simulink model "vertical_smm_with_lqr_2d"  (R2015a)
settings: Solver=FixedStepDiscrete  StartTime=0.0  StopTime=inf  FixedStep=sample_time  RelTol=1e-3
undefined symbols (not defined in the file or in its folder): A_kalman_fourbar_gear, A_kalman_transverse, A_kalman_vertical, A_lpf_dtau, A_lpf_leg_spring, B1_lpf_dtau, B1_lpf_leg_spring, B2_lpf_dtau, B2_lpf_leg_spring, B_dx_versus_x0, B_kalman_fourbar_gear, B_kalman_transverse, B_kalman_vertical, backwards_K_sag_of_t, boom_mount_angle, C_kalman_fourbar_gear, C_kalman_transverse, C_kalman_vertical, com_leg_motor, com_torso, contact_threshold, control_start_time, d_vertical_boom_com_offset, d_vertical_com, desired_com_forward_velocity, desired_torso_angle, Discrete, fcut_contact, forward_dx, forward_dx_of_dxstar, forward_velocity_target_step, forward_x, forward_x_of_dxstar, g, h_boom, HIP_MTR_MAX_CONT_TORQUE, i_robot, initial_dx_estimate, initial_dy_estimate, initial_dz_estimate, initial_z_estimate, j_leg, j_motor, j_segments, k_LQR_vertical, k_sea, k_vertical_winch, kalman_load_to_deflect_transmission, kalman_stance_slip_threshold, kd_lateral, kd_motor, kp_lateral, kp_motor, l_boom_projected, l_retract_delta, l_retract_swing_max, l_retract_swing_min, l_seg, lambda1, lambda2 ... (+60)
libraries: simulink x9, ctrlSharedLib x7
(part 2 of 4)

== system vertical_smm_with_lqr_2d/Control/Behavior Control/R Leg Calculator ==
  Front [rad rad/s] : Inport
  Back [rad rad/s] : Inport  Port=2
  Demux1 : Demux  Outputs=2
  Gain1 : Gain  Gain=2*l_seg
  Gain2 : Gain  Gain=l_seg
  Gain3 : Gain  Gain=-1
  Gain4 : Gain  Gain=0.5
  Gain5 : Gain  Gain=0.5
  Gain6 : Gain  Gain=2
  Mux1 : Mux  Inputs=2
  Product : Product  RndMeth=Zero
  Sum4 : Sum  Inputs=+|+
  Sum5 : Sum  Inputs=+|-
  Trigonometric Function : Trigonometry  Operator=cos
  Trigonometric Function1 : Trigonometry
  "Leg Length [m m/s] " : Outport
  Leg Angle [rad rad/s] : Outport  Port=2
  Leg Splay [rad rad/s] : Outport  Port=3
  w [m] : Outport  Port=4
  wires:
  Gain5/1 -> Leg Angle [rad rad/s]/1
  Sum4/1 -> Gain5/1
  Mux1/1 -> "Leg Length [m m/s] "/1
  Sum5/1 -> Demux1/1, Leg Splay [rad rad/s]/1
  Gain2/1 -> Gain6/1, Product/1
  Demux1/1 -> Gain4/1
  Gain3/1 -> Product/2
  Demux1/2 -> Gain3/1
  Back [rad rad/s]/1 -> Sum5/1, Sum4/1
  Front [rad rad/s]/1 -> Sum4/2, Sum5/2
  Product/1 -> Mux1/2
  Trigonometric Function1/1 -> Gain2/1
  Gain1/1 -> Mux1/1
  Trigonometric Function/1 -> Gain1/1
  Gain4/1 -> Trigonometric Function/1, Trigonometric Function1/1
  Gain6/1 -> w [m]/1

== system vertical_smm_with_lqr_2d/Control/Behavior Control/Secondary Leg Behavior ==
  note: Mirror the primary
      | leg motion
  note: Position control the
      | individual four bar segments
  note: Convert to
      | four-bar angles
  Secondary Back Gear [rad rad/s] : Inport
  Secondary Front Gear [rad rad/s] : Inport  Port=2
  Torso Pitch [rad rad/s] : Inport  Port=3
  Right/Left Secondary [1/0] : Inport  Port=4
  Primary Leg Angle [rad rad/s] : Inport  Port=5
  Primary Leg Length [m m/s] : Inport  Port=6
  Avoid Hitting Mechanical Limits : MATLAB Function  TreatAsAtomicUnit=on
  Back/Front Motor PD : Subsystem
  Constant4 : Constant  Value=0
  Constant5 : Constant  Value=0  OutDataTypeStr=boolean
  Demux{1..3,5} (4 alike) : Demux  Outputs=2
  Demux6 : Demux  Outputs=6
  Fcn2 : Fcn  Expr=2*pi-u(1)
  Mirrored Leg Length Target : MATLAB Function  TreatAsAtomicUnit=on
  Mux{1..4,7,11} (6 alike) : Mux  Inputs=2
  Mux5 : Mux  Inputs=3
  Mux6 : Mux  Inputs=3
  Sum1 : Sum  Inputs=++|
  Virtual Leg to Four Bar : MATLAB Function  TreatAsAtomicUnit=on
  k_virtual6 : Gain  Gain=-1
  two_pole_filter : DiscreteTransferFcn  Numerator=[A_lpf_leg_spring 0 0]  Denominator=[1 B1_lpf_leg_spring B2_lpf_leg_spring]  SampleTime=sample_time
  Secondary Back/Front Motor Torque [Nm Nm] : Outport
  Secondary Force or Position Control [1/0] : Outport  Port=2
  wires:
  Constant5/1 -> Secondary Force or Position Control [1/0]/1
  Back/Front Motor PD/1(Commanded Torque [Nm] [back front]) -> Secondary Back/Front Motor Torque [Nm Nm]/1
  Demux5/2 -> k_virtual6/1
  Demux5/1 -> Fcn2/1
  Primary Leg Angle [rad rad/s]/1 -> two_pole_filter/1
  Mirrored Leg Length Target/2(dl_leg) -> Mux5/2
  Mirrored Leg Length Target/3(ddl_leg) -> Mux5/3
  Mirrored Leg Length Target/1(l_leg) -> Mux5/1
  Constant4/1 -> Mux6/3
  k_virtual6/1 -> Mux6/2
  Fcn2/1 -> Mux6/1
  Mux7/1 -> Demux6/1
  Torso Pitch [rad rad/s]/1 -> Sum1/1
  Mux5/1 -> Mux7/1
  Mux6/1 -> Mux7/2
  Virtual Leg to Four Bar/1(back) -> Avoid Hitting Mechanical Limits/1(back_desired)
  Virtual Leg to Four Bar/2(dback) -> Avoid Hitting Mechanical Limits/2(dback_desired)
  Virtual Leg to Four Bar/3(ddback) -> Avoid Hitting Mechanical Limits/3(ddback_desired)
  Virtual Leg to Four Bar/4(front) -> Avoid Hitting Mechanical Limits/4(front_desired)
  Virtual Leg to Four Bar/5(dfront) -> Avoid Hitting Mechanical Limits/5(dfront_desired)
  Virtual Leg to Four Bar/6(ddfront) -> Avoid Hitting Mechanical Limits/6(ddfront_desired)
  Demux6/1 -> Virtual Leg to Four Bar/1(l_leg)
  Demux6/2 -> Virtual Leg to Four Bar/2(dl_leg)
  Demux6/3 -> Virtual Leg to Four Bar/3(ddl_leg)
  Demux6/4 -> Virtual Leg to Four Bar/4(phi)
  Demux6/5 -> Virtual Leg to Four Bar/5(dphi)
  Demux6/6 -> Virtual Leg to Four Bar/6(ddphi)
  Mux11/1 -> Back/Front Motor PD/5(Measured Velocity [rad/s] [back front])
  Demux2/2 -> Mux11/2
  Mux4/1 -> Back/Front Motor PD/4(Measured Position [rad] [back front])
  Mux1/1 -> Back/Front Motor PD/1(Desired Position [rad] [back front])
  Right/Left Secondary [1/0]/1 -> Back/Front Motor PD/6(Right/Left Leg [1/0])
  Demux3/2 -> Mux11/1
  Demux3/1 -> Mux4/1
  Avoid Hitting Mechanical Limits/2(front_cmd) -> Mux1/2
  Avoid Hitting Mechanical Limits/1(back_cmd) -> Mux1/1
  Demux2/1 -> Mux4/2
  Secondary Front Gear [rad rad/s]/1 -> Demux2/1
  Secondary Back Gear [rad rad/s]/1 -> Demux3/1
  Avoid Hitting Mechanical Limits/3(dback_cmd) -> Mux2/1
  Avoid Hitting Mechanical Limits/4(dfront_cmd) -> Mux2/2
  Avoid Hitting Mechanical Limits/5(ddback_cmd) -> Mux3/1
  Avoid Hitting Mechanical Limits/6(ddfront_cmd) -> Mux3/2
  Mux2/1 -> Back/Front Motor PD/2(Desired Velocity [rad/s] [back front])
  Mux3/1 -> Back/Front Motor PD/3(Desired Acceleration [rad/s^2] [back front])
  two_pole_filter/1 -> Sum1/2
  Sum1/1 -> Demux5/1
  Demux1/1 -> Mirrored Leg Length Target/1(primary_l_leg)
  Demux1/2 -> Mirrored Leg Length Target/2(primary_dl_leg)
  Primary Leg Length [m m/s]/1 -> Demux1/1

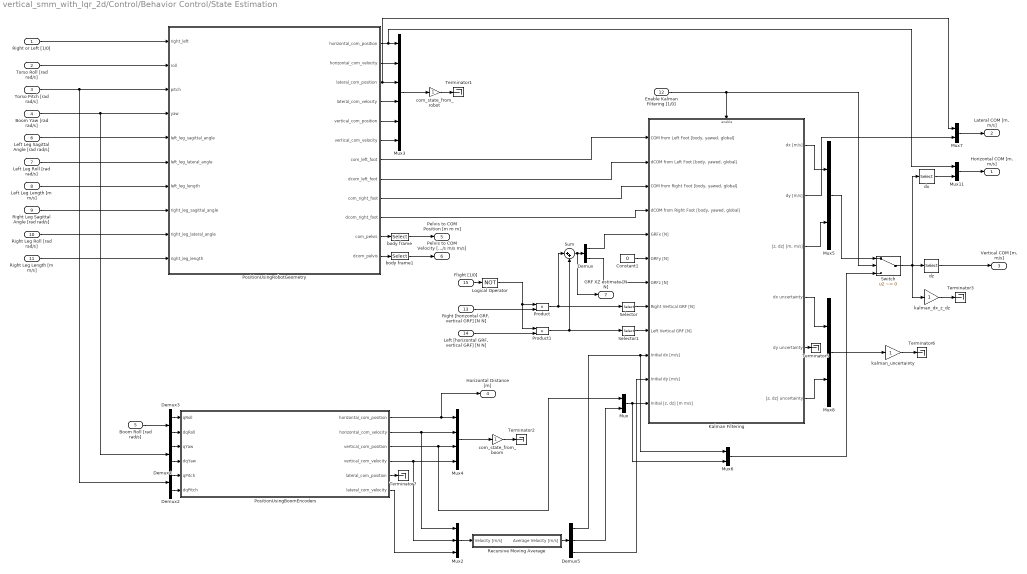
== system vertical_smm_with_lqr_2d/Control/Behavior Control/State Estimation ==
  Right or Left [1/0] : Inport
  Torso Roll [rad rad/s] : Inport  Port=2
  Torso Pitch [rad rad/s] : Inport  Port=3
  Boom Yaw [rad rad/s] : Inport  Port=4
  Boom Roll [rad rad/s] : Inport  Port=5
  Left Leg Sagittal Angle [rad rad/s] : Inport  Port=6
  Left Leg Roll [rad rad/s] : Inport  Port=7
  Left Leg Length [m m/s] : Inport  Port=8
  Right Leg Sagittal Angle [rad rad/s] : Inport  Port=9
  Right Leg Roll [rad rad/s] : Inport  Port=10
  Right Leg Length [m m/s] : Inport  Port=11
  Enable Kalman Filtering [1/0] : Inport  Port=12
  "Right [horizontal GRF, vertical GRF] [N N]" : Inport  Port=13
  "Left [horizontal GRF, vertical GRF] [N N]" : Inport  Port=14
  Flight [1/0] : Inport  Port=15
  Constant1 : Constant  Value=0
  Demux{,2..4} (4 alike) : Demux  Outputs=2
  Demux5 : Demux  Outputs=3
  Kalman Filtering : Subsystem
  Logical Operator : Logic  Operator=NOT  AllPortsSameDT=off  OutDataTypeStr=boolean
  Mux{,5..8,11} (6 alike) : Mux  Inputs=2
  Mux2 : Mux  Inputs=3
  Mux3 : Mux  Inputs=6
  Mux4 : Mux
  PositionUsingBoomEncoders : MATLAB Function  TreatAsAtomicUnit=on
  PositionUsingRobotGeometry : MATLAB Function  TreatAsAtomicUnit=on
  Product : Product
  Product1 : Product
  Recursive Moving Average : Subsystem
  Selector : Selector  InputPortWidth=2  Indices=[2]
  Selector1 : Selector  InputPortWidth=2  Indices=[2]
  Sum : Sum  Inputs=|++
  Switch : Switch  Criteria=u2 ~= 0
  Terminator{1..3,5..7} (6 alike) : Terminator
  body frame : Selector  InputPortWidth=9  Indices=[1 2 3]
  body frame1 : Selector  InputPortWidth=9  Indices=[1 2 3]
  com_state_from_boom : Gain
  com_state_from_robot : Gain
  dx : Selector  InputPortWidth=3  Indices=[1]
  dz : Selector  InputPortWidth=3  Indices=[2 3]
  kalman_dx_z_dz : Gain
  kalman_uncertainty : Gain
  "Horizontal COM [m, m/s]" : Outport
  "Lateral COM [m, m/s]" : Outport  Port=2
  "Vertical COM [m, m/s]" : Outport  Port=3
  Horizontal Distance [m] : Outport  Port=4
  Pelvis to COM Position [m m m] : Outport  Port=5
  Pelvis to COM Velocity [m/s m/s m/s] : Outport  Port=6
  GRF XZ estimate [N N] : Outport  Port=7
  wires:
  com_state_from_boom/1 -> Terminator2/1
  Kalman Filtering/1(dx [m/s]) -> Mux5/1
  Demux2/1 -> PositionUsingBoomEncoders/5(qPitch)
  Demux2/2 -> PositionUsingBoomEncoders/6(dqPitch)
  Mux3/1 -> com_state_from_robot/1
  com_state_from_robot/1 -> Terminator1/1
  PositionUsingRobotGeometry/1(horizontal_com_position) -> Mux3/1, Mux11/1
  PositionUsingBoomEncoders/1(horizontal_com_position) -> Horizontal Distance [m]/1, Mux4/1
  PositionUsingBoomEncoders/3(vertical_com_position) -> Mux/1, Mux4/3
  PositionUsingBoomEncoders/4(vertical_com_velocity) -> Mux2/2, Mux4/4
  Mux4/1 -> com_state_from_boom/1
  Left Leg Sagittal Angle [rad rad/s]/1 -> PositionUsingRobotGeometry/5(left_leg_sagittal_angle)
  Left Leg Roll [rad rad/s]/1 -> PositionUsingRobotGeometry/6(left_leg_lateral_angle)
  Left Leg Length [m m/s]/1 -> PositionUsingRobotGeometry/7(left_leg_length)
  Right Leg Sagittal Angle [rad rad/s]/1 -> PositionUsingRobotGeometry/8(right_leg_sagittal_angle)
  Right Leg Roll [rad rad/s]/1 -> PositionUsingRobotGeometry/9(right_leg_lateral_angle)
  Right Leg Length [m m/s]/1 -> PositionUsingRobotGeometry/10(right_leg_length)
  Right or Left [1/0]/1 -> PositionUsingRobotGeometry/1(right_left)
  Torso Roll [rad rad/s]/1 -> PositionUsingRobotGeometry/2(roll)
  Boom Yaw [rad rad/s]/1 -> Demux4/1, PositionUsingRobotGeometry/4(yaw)
  Torso Pitch [rad rad/s]/1 -> Demux2/1, PositionUsingRobotGeometry/3(pitch)
  Demux3/2 -> PositionUsingBoomEncoders/2(dqRoll)
  Demux3/1 -> PositionUsingBoomEncoders/1(qRoll)
  Boom Roll [rad rad/s]/1 -> Demux3/1
  Demux4/1 -> PositionUsingBoomEncoders/3(qYaw)
  Demux4/2 -> PositionUsingBoomEncoders/4(dqYaw)
  PositionUsingRobotGeometry/7(com_left_foot) -> Kalman Filtering/1("COM from Left Foot [body, yawed, global]")
  PositionUsingRobotGeometry/8(dcom_left_foot) -> Kalman Filtering/2("dCOM from Left Foot [body, yawed, global]")
  PositionUsingRobotGeometry/9(com_right_foot) -> Kalman Filtering/3("COM from Right Foot [body, yawed, global]")
  PositionUsingRobotGeometry/10(dcom_right_foot) -> Kalman Filtering/4("dCOM from Right Foot [body, yawed, global]")
  Kalman Filtering/2(dy [m/s]) -> Mux7/2
  Kalman Filtering/3("[z, dz] [m, m/s]") -> Mux5/2
  Mux2/1 -> Recursive Moving Average/1(Velocity [m/s])
  dx/1 -> Mux11/2
  Mux5/1 -> Switch/1
  Constant1/1 -> Kalman Filtering/6(GRFy [N])
  Recursive Moving Average/1(Average Velocity [m/s]) -> Demux5/1
  Mux/1 -> Mux6/2, Kalman Filtering/12("Initial [z, dz] [m m/s]")
  Demux5/2 -> Mux/2
  PositionUsingBoomEncoders/2(horizontal_com_velocity) -> Mux2/1, Mux4/2
  Selector/1 -> Kalman Filtering/8(Right Vertical GRF [N])
  Selector1/1 -> Kalman Filtering/9(Left Vertical GRF [N])
  Product1/1 -> Sum/2, Selector1/1
  Product/1 -> Sum/1, Selector/1
  Sum/1 -> GRF XZ estimate [N N]/1, Demux/1
  Enable Kalman Filtering [1/0]/1 -> Switch/2, Kalman Filtering/Enable
  kalman_dx_z_dz/1 -> Terminator3/1
  Demux5/1 -> Mux6/1, Kalman Filtering/10(Initial dx [m/s])
  Demux/1 -> Kalman Filtering/5(GRFx [N])
  Demux/2 -> Kalman Filtering/7(GRFz [N])
  Flight [1/0]/1 -> Logical Operator/1
  "Right [horizontal GRF, vertical GRF] [N N]"/1 -> Product/2
  Logical Operator/1 -> Product1/1, Product/1
  "Left [horizontal GRF, vertical GRF] [N N]"/1 -> Product1/2
  Kalman Filtering/4(dx uncertainty) -> Mux8/1
  Kalman Filtering/6("[z, dz] uncertainty") -> Mux8/2
  Kalman Filtering/5(dy uncertainty) -> Terminator5/1
  kalman_uncertainty/1 -> Terminator6/1
  Mux8/1 -> kalman_uncertainty/1
  PositionUsingRobotGeometry/12(dcom_pelvis) -> body frame1/1
  PositionUsingRobotGeometry/11(com_pelvis) -> body frame/1
  Mux11/1 -> "Horizontal COM [m, m/s]"/1
  body frame/1 -> Pelvis to COM Position [m m m]/1
  body frame1/1 -> Pelvis to COM Velocity [m/s m/s m/s]/1
  PositionUsingRobotGeometry/6(vertical_com_velocity) -> Mux3/6
  PositionUsingRobotGeometry/5(vertical_com_position) -> Mux3/5
  PositionUsingRobotGeometry/4(lateral_com_velocity) -> Mux3/4
  PositionUsingRobotGeometry/3(lateral_com_position) -> Mux3/3, Mux7/1
  PositionUsingRobotGeometry/2(horizontal_com_velocity) -> Mux3/2
  Mux6/1 -> Switch/3
  dz/1 -> "Vertical COM [m, m/s]"/1
  Switch/1 -> dx/1, dz/1, kalman_dx_z_dz/1
  Mux7/1 -> "Lateral COM [m, m/s]"/1
  PositionUsingBoomEncoders/5(lateral_com_position) -> Terminator7/1
  PositionUsingBoomEncoders/6(lateral_com_velocity) -> Mux2/3
  Demux5/3 -> Kalman Filtering/11(Initial dy [m/s])

== system vertical_smm_with_lqr_2d/Control/Behavior Control/Torque Distribution Left ==
  Leg Torque [Nm] : Inport
  Leg Force [N] : Inport  Port=2
  w [m] : Inport  Port=3
  Gain : Gain  Gain=0.5
  Gain1 : Gain  Gain=0.5
  Motor Torque Saturation Optimization : MATLAB Function  TreatAsAtomicUnit=on
  Product : Product  RndMeth=Zero
  Sum : Sum  Inputs=|++
  Sum1 : Sum  Inputs=+-|
  Back Torque [Nm] : Outport
  Front Torque [Nm] : Outport  Port=2
  wires:
  Gain/1 -> Motor Torque Saturation Optimization/1(x1s)
  Gain1/1 -> Motor Torque Saturation Optimization/2(x2s)
  Product/1 -> Gain1/1
  Leg Force [N]/1 -> Product/1
  Motor Torque Saturation Optimization/2(t2) -> Sum/2, Sum1/2
  w [m]/1 -> Product/2
  Motor Torque Saturation Optimization/1(t1) -> Sum1/1, Sum/1
  Sum/1 -> Front Torque [Nm]/1
  Leg Torque [Nm]/1 -> Gain/1
  Sum1/1 -> Back Torque [Nm]/1

== system vertical_smm_with_lqr_2d/Control/Behavior Control/Torque Distribution Right ==
  Leg Torque [Nm] : Inport
  Leg Force [N] : Inport  Port=2
  w [m] : Inport  Port=3
  Gain : Gain  Gain=0.5
  Gain1 : Gain  Gain=0.5
  Motor Torque Saturation Optimization : MATLAB Function  TreatAsAtomicUnit=on
  Product : Product  RndMeth=Zero
  Sum : Sum  Inputs=|++
  Sum1 : Sum  Inputs=+-|
  Back Torque [Nm] : Outport
  Front Torque [Nm] : Outport  Port=2
  wires:
  Sum1/1 -> Back Torque [Nm]/1
  Leg Torque [Nm]/1 -> Gain/1
  Sum/1 -> Front Torque [Nm]/1
  Motor Torque Saturation Optimization/1(t1) -> Sum/1, Sum1/1
  w [m]/1 -> Product/2
  Motor Torque Saturation Optimization/2(t2) -> Sum1/2, Sum/2
  Leg Force [N]/1 -> Product/1
  Product/1 -> Gain1/1
  Gain1/1 -> Motor Torque Saturation Optimization/2(x2s)
  Gain/1 -> Motor Torque Saturation Optimization/1(x1s)

== system vertical_smm_with_lqr_2d/Control/Behavior Control/dtau_des ==
  x : Inport
  Gain1 : Gain  Gain=1/sample_time
  difference : simulink/Discrete/Difference  ICPrevInput=0.0  InputProcessing=Inherited  OutMin=[]  OutMax=[]  OutDataType=fixdt(1, 16)  OutScaling=2^-10  DoSatur=off
  two_pole_filter : DiscreteTransferFcn  Numerator=[A_lpf_dtau 0 0]  Denominator=[1 B1_lpf_dtau B2_lpf_dtau]  SampleTime=sample_time
  dx/dt : Outport
  wires:
  two_pole_filter/1 -> dx/dt/1
  x/1 -> Gain1/1
  difference/1 -> two_pole_filter/1
  Gain1/1 -> difference/1

== system vertical_smm_with_lqr_2d/Control/Behavior Control/Force Estimation/Horizontal GRF ==
  Axial Force [N] : Inport
  Orthogonal Force [N] : Inport  Port=2
  Torso Pitch [rad] : Inport  Port=3
  Leg Angle [rad] : Inport  Port=4
  Gain : Gain  Gain=-1
  Gain1 : Gain  Gain=-1
  Product : Product
  Product1 : Product
  Sum : Sum  Inputs=++|
  Sum1 : Sum  Inputs=+|+
  Trigonometric Function : Trigonometry
  Trigonometric Function1 : Trigonometry  Operator=cos
  Horizontal Force [N] : Outport
  wires:
  Product1/1 -> Gain/1
  Sum1/1 -> Horizontal Force [N]/1
  Trigonometric Function1/1 -> Product1/2
  Orthogonal Force [N]/1 -> Product1/1
  Axial Force [N]/1 -> Product/1
  Leg Angle [rad]/1 -> Sum/2
  Torso Pitch [rad]/1 -> Sum/1
  Trigonometric Function/1 -> Product/2
  Sum/1 -> Trigonometric Function/1, Trigonometric Function1/1
  Product/1 -> Gain1/1
  Gain/1 -> Sum1/2
  Gain1/1 -> Sum1/1

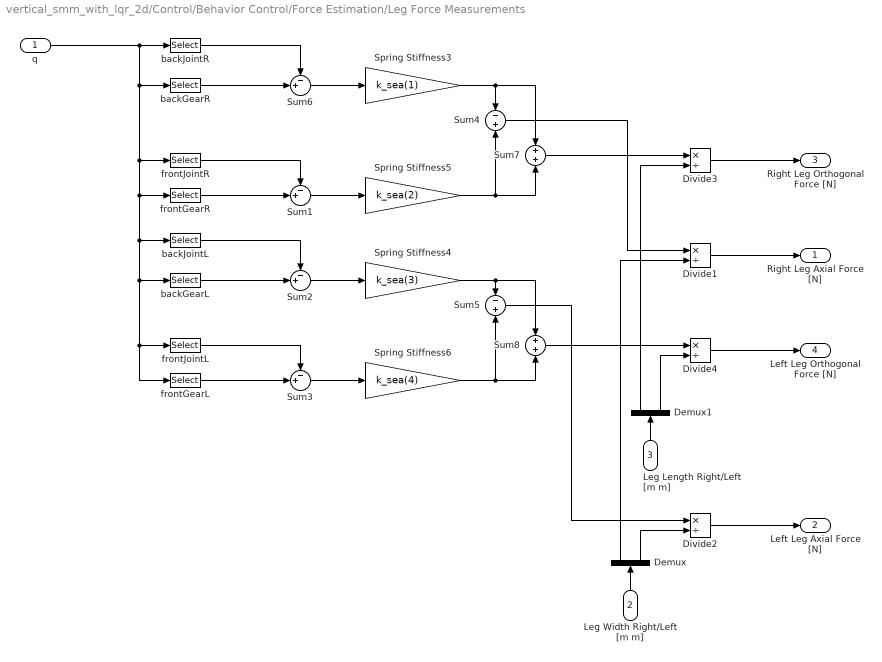
== system vertical_smm_with_lqr_2d/Control/Behavior Control/Force Estimation/Leg Force Measurements ==
  q : Inport
  Leg Width Right/Left [m m] : Inport  Port=2
  Leg Length Right/Left [m m] : Inport  Port=3
  Demux : Demux  Outputs=2
  Demux1 : Demux  Outputs=2
  Divide{1..4} (4 alike) : Product  Inputs=*/
  Spring Stiffness3 : Gain  Gain=k_sea(1)
  Spring Stiffness4 : Gain  Gain=k_sea(3)
  Spring Stiffness5 : Gain  Gain=k_sea(2)
  Spring Stiffness6 : Gain  Gain=k_sea(4)
  Sum{1..3,6} (4 alike) : Sum  Inputs=-+|
  Sum4 : Sum  Inputs=-|+
  Sum5 : Sum  Inputs=-|+
  Sum7 : Sum  Inputs=+|+
  Sum8 : Sum  Inputs=+|+
  backGearL : Selector  InputPortWidth=13  Indices=[6]
  backGearR : Selector  InputPortWidth=13  Indices=[2]
  backJointL : Selector  InputPortWidth=13  Indices=[5]
  backJointR : Selector  InputPortWidth=13  Indices=[1]
  frontGearL : Selector  InputPortWidth=13  Indices=[8]
  frontGearR : Selector  InputPortWidth=13  Indices=[4]
  frontJointL : Selector  InputPortWidth=13  Indices=[7]
  frontJointR : Selector  InputPortWidth=13  Indices=[3]
  Right Leg Axial Force [N] : Outport
  Left Leg Axial Force [N] : Outport  Port=2
  Right Leg Orthogonal Force [N] : Outport  Port=3
  Left Leg Orthogonal Force [N] : Outport  Port=4
  wires:
  Sum3/1 -> Spring Stiffness6/1
  Sum2/1 -> Spring Stiffness4/1
  backJointL/1 -> Sum2/1
  frontGearL/1 -> Sum3/2
  frontJointL/1 -> Sum3/1
  backGearL/1 -> Sum2/2
  Sum6/1 -> Spring Stiffness3/1
  Sum1/1 -> Spring Stiffness5/1
  backJointR/1 -> Sum6/1
  frontGearR/1 -> Sum1/2
  frontJointR/1 -> Sum1/1
  backGearR/1 -> Sum6/2
  q/1 -> backGearR/1, backJointL/1, frontJointL/1, frontGearL/1, backGearL/1, frontGearR/1, frontJointR/1, backJointR/1
  Spring Stiffness3/1 -> Sum7/1, Sum4/1
  Spring Stiffness5/1 -> Sum7/2, Sum4/2
  Spring Stiffness6/1 -> Sum8/2, Sum5/2
  Sum4/1 -> Divide1/1
  Sum5/1 -> Divide2/1
  Leg Width Right/Left [m m]/1 -> Demux/1
  Demux/1 -> Divide1/2
  Demux/2 -> Divide2/2
  Divide1/1 -> Right Leg Axial Force [N]/1
  Divide2/1 -> Left Leg Axial Force [N]/1
  Spring Stiffness4/1 -> Sum8/1, Sum5/1
  Sum7/1 -> Divide3/1
  Sum8/1 -> Divide4/1
  Divide3/1 -> Right Leg Orthogonal Force [N]/1
  Divide4/1 -> Left Leg Orthogonal Force [N]/1
  Demux1/1 -> Divide3/2
  Demux1/2 -> Divide4/2
  Leg Length Right/Left [m m]/1 -> Demux1/1

== system vertical_smm_with_lqr_2d/Control/Behavior Control/Force Estimation/Vertical GRF ==
  Axial Force [N] : Inport
  Orthogonal Force [N] : Inport  Port=2
  Torso Pitch [rad] : Inport  Port=3
  Leg Angle [rad] : Inport  Port=4
  Gain : Gain  Gain=-1
  Product : Product
  Product1 : Product
  Sum : Sum  Inputs=++|
  Sum1 : Sum  Inputs=+|+
  Trigonometric Function : Trigonometry  Operator=cos
  Trigonometric Function1 : Trigonometry
  Vertical Force [N] : Outport
  wires:
  Gain/1 -> Sum1/1
  Sum/1 -> Trigonometric Function1/1, Trigonometric Function/1
  Product/1 -> Gain/1
  Trigonometric Function/1 -> Product/2
  Torso Pitch [rad]/1 -> Sum/1
  Leg Angle [rad]/1 -> Sum/2
  Axial Force [N]/1 -> Product/1
  Orthogonal Force [N]/1 -> Product1/1
  Trigonometric Function1/1 -> Product1/2
  Sum1/1 -> Vertical Force [N]/1
  Product1/1 -> Sum1/2

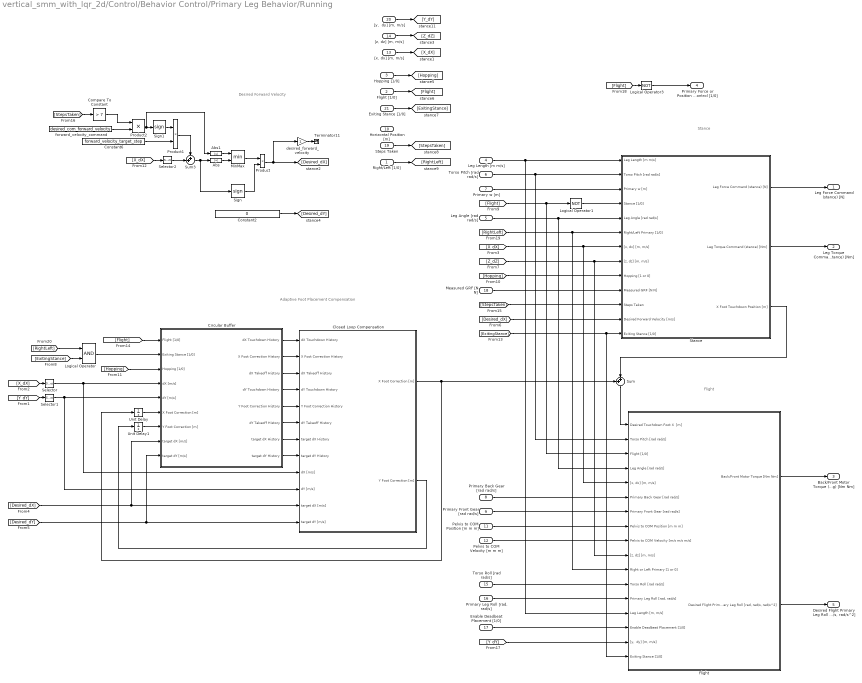
== system vertical_smm_with_lqr_2d/Control/Behavior Control/Primary Leg Behavior/Running ==
  note: Stance
  note: Flight
  note: Adaptive Foot Placement Compensation
  note: Desired Forward Velocity
  Right/Left [1/0] : Inport
  Flight [1/0] : Inport  Port=2
  Hopping [1/0] : Inport  Port=3
  Leg Length [m m/s] : Inport  Port=4
  Leg Angle [rad rad/s] : Inport  Port=5
  Torso Pitch [rad rad/s] : Inport  Port=6
  Primary w [m] : Inport  Port=7
  Primary Back Gear [rad rad/s] : Inport  Port=8
  Primary Front Gear [rad rad/s] : Inport  Port=9
  Horizontal Position [m] : Inport  Port=10
  Pelvis to COM Position [m m m] : Inport  Port=11
  Pelvis to COM Velocity [m m m] : Inport  Port=12
  "[x, dx] [m, m/s]" : Inport  Port=13
  "[z, dz] [m, m/s]" : Inport  Port=14
  Torso Roll [rad rad/s] : Inport  Port=15
  "Primary Leg Roll [rad, rad/s]" : Inport  Port=16
  Enable Deadbeat Placement [1/0] : Inport  Port=17
  Measured GRF [N N] : Inport  Port=18
  Steps Taken : Inport  Port=19
  "[y,  dy] [m, m/s]" : Inport  Port=20
  Exiting Stance [1/0] : Inport  Port=21
  Abs : Abs
  Abs1 : Abs
  Circular Buffer : Subsystem
  Closed Loop Compensation : Subsystem
  Compare To Constant : simulink/Logic and Bit Operations/Compare To Constant  relop=>  const=7  OutDataTypeStr=boolean
  Constant2 : Constant  Value=0
  Constant6 : Constant  Value=forward_velocity_target_step
  Flight : Subsystem
  Logical Operator : Logic  AllPortsSameDT=off  OutDataTypeStr=boolean
  Logical Operator1 : Logic  Operator=NOT  AllPortsSameDT=off  OutDataTypeStr=boolean
  Logical Operator3 : Logic  Operator=NOT  AllPortsSameDT=off  OutDataTypeStr=boolean
  MinMax : MinMax  Inputs=2
  Product : Product
  Product1 : Product
  Product2 : Product
  Selector : Selector  InputPortWidth=2  Indices=[2]
  Selector1 : Selector  InputPortWidth=2  Indices=[2]
  Selector2 : Selector  InputPortWidth=2  Indices=[2]
  Sign : Signum
  Sign1 : Signum
  Stance : Subsystem
  Sum : Sum  Inputs=++|
  Sum3 : Sum  Inputs=++|
  Terminator11 : Terminator
  Unit Delay : UnitDelay  SampleTime=-1
  Unit Delay1 : UnitDelay  SampleTime=-1
  desired_forward_velocity : Gain
  forward_velocity_command : Constant  Description=xPCTag(1) = forward_velocity_command;  Value=desired_com_forward_velocity
  Leg Force Command (stance) [N] : Outport
  Leg Torque Command (stance) [Nm] : Outport  Port=2
  Back/Front Motor Torque (swing) [Nm Nm] : Outport  Port=3
  Primary Force or Position Control [1/0] : Outport  Port=4  OutDataTypeStr=boolean
  "Desired Flight Primary Leg Roll [rad, rad/s, rad/s^2]" : Outport  Port=5
  wires:
  Leg Length [m m/s]/1 -> Stance/1(Leg Length [m m/s]), Flight/14("Leg Length [m, m/s]")
  Primary w [m]/1 -> Stance/3(Primary w [m])
  Stance/1(Leg Force Command (stance) [N]) -> Leg Force Command (stance) [N]/1
  Stance/2(Leg Torque Command (stance) [Nm]) -> Leg Torque Command (stance) [Nm]/1
  Torso Pitch [rad rad/s]/1 -> Flight/2(Torso Pitch [rad rad/s]), Stance/2(Torso Pitch [rad rad/s])
  [Hopping] -> Stance/9(Hopping [1 or 0])
  [X_dX] -> Flight/5("[x, dx] [m, m/s]"), Stance/7("[x, dx] [m, m/s]")
  [RightLeft] -> Flight/11(Right or Left Primary [1 or 0]), Stance/6(Right/Left Primary [1/0])
  Primary Back Gear [rad rad/s]/1 -> Flight/6(Primary Back Gear [rad rad/s])
  Primary Front Gear [rad rad/s]/1 -> Flight/7(Primary Front Gear [rad rad/s])
  Leg Angle [rad rad/s]/1 -> Flight/4(Leg Angle [rad rad/s]), Stance/5(Leg Angle [rad rad/s])
  Flight/1(Back/Front Motor Torque [Nm Nm]) -> Back/Front Motor Torque (swing) [Nm Nm]/1
  Logical Operator1/1 -> Stance/4(Stance [1/0])
  Pelvis to COM Position [m m m]/1 -> Flight/8(Pelvis to COM Position [m m m])
  [Z_dZ] -> Flight/10("[z, dz] [m, m/s]"), Stance/8("[z, dz] [m, m/s]")
  Pelvis to COM Velocity [m m m]/1 -> Flight/9(Pelvis to COM Velocity [m/s m/s m/s])
  Torso Roll [rad rad/s]/1 -> Flight/12(Torso Roll [rad rad/s])
  "Primary Leg Roll [rad, rad/s]"/1 -> Flight/13("Primary Leg Roll [rad, rad/s]")
  Enable Deadbeat Placement [1/0]/1 -> Flight/15(Enable Deadbeat Placement [1/0])
  Flight/2("Desired Flight Primary Leg Roll [rad, rad/s, rad/s^2]") -> "Desired Flight Primary Leg Roll [rad, rad/s, rad/s^2]"/1
  Measured GRF [N N]/1 -> Stance/10(Measured GRF [N N])
  [StepsTaken] -> Stance/11(Steps Taken)
  [Y_dY] -> Flight/16("[y,  dy] [m, m/s]")
  Circular Buffer/1("dX Touchdown History ") -> Closed Loop Compensation/1(dX Touchdown History)
  Circular Buffer/2(X Foot Correction History) -> Closed Loop Compensation/2(X Foot Correction History)
  Circular Buffer/3(dX Takeoff History) -> Closed Loop Compensation/3(dX Takeoff History)
  Circular Buffer/4("dY Touchdown History ") -> Closed Loop Compensation/4(dY Touchdown History)
  Circular Buffer/5(Y Foot Correction History) -> Closed Loop Compensation/5(Y Foot Correction History)
  Circular Buffer/6(dY Takeoff History) -> Closed Loop Compensation/6(dY Takeoff History)
  Circular Buffer/8(target dY History) -> Closed Loop Compensation/8(target dY History)
  Circular Buffer/7(target dX History) -> Closed Loop Compensation/7(target dX History)
  [Desired_dX] -> Circular Buffer/8(target dX [m/s]), Closed Loop Compensation/11(target dX [m/s])
  [Desired_dY] -> Circular Buffer/9(target dY [m/s]), Closed Loop Compensation/12("target dY [m/s] ")
  Stance/3(X Foot Touchdown Position [m]) -> Sum/2
  Sum/1 -> Flight/1(Desired Touchdown Foot X  [m])
  Closed Loop Compensation/1(X Foot Correction [m]) -> Unit Delay/1, Sum/1
  Selector1/1 -> Closed Loop Compensation/10(dY [m/s]), Circular Buffer/5(dY [m/s])
  Selector/1 -> Circular Buffer/4(dX [m/s]), Closed Loop Compensation/9(dX [m/s])
  Unit Delay1/1 -> Circular Buffer/7(Y Foot Correction [m])
  Unit Delay/1 -> Circular Buffer/6(X Foot Correction [m])
  Closed Loop Compensation/2(Y Foot Correction [m]) -> Unit Delay1/1
  "[x, dx] [m, m/s]"/1 -> [X_dX]
  "[z, dz] [m, m/s]"/1 -> [Z_dZ]
  "[y,  dy] [m, m/s]"/1 -> [Y_dY]
  [X_dX] -> Selector/1
  [Y_dY] -> Selector1/1
  MinMax/1 -> Product/1
  Constant2/1 -> [Desired_dY]
  [Desired_dX] -> Stance/12(Desired Forward Velocity [m/s])
  Flight [1/0]/1 -> [Flight]
  [Flight] -> Logical Operator1/1, Flight/3(Flight [1/0])
  Hopping [1/0]/1 -> [Hopping]
  Sum3/1 -> Abs/1, Sign/1
  Selector2/1 -> Sum3/2
  [X_dX] -> Selector2/1
  Sign/1 -> Product/2
  Abs/1 -> MinMax/2
  Product2/1 -> Abs1/1, Sign1/1
  Sign1/1 -> Product1/1
  Constant6/1 -> Product1/2
  Product1/1 -> Sum3/1
  Exiting Stance [1/0]/1 -> [ExitingStance]
  [ExitingStance] -> Flight/17(Exiting Stance [1/0]), Stance/13(Exiting Stance [1/0])
  [Hopping] -> Circular Buffer/3(Hopping [1/0])
  Logical Operator/1 -> Circular Buffer/2(Exiting Stance [1/0])
  [Flight] -> Circular Buffer/1(Flight [1/0])
  [Flight] -> Logical Operator3/1
  Logical Operator3/1 -> Primary Force or Position Control [1/0]/1
  Product/1 -> [Desired_dX], desired_forward_velocity/1
  desired_forward_velocity/1 -> Terminator11/1
  Abs1/1 -> MinMax/1
  Steps Taken/1 -> [StepsTaken]
  [StepsTaken] -> Compare To Constant/1
  forward_velocity_command/1 -> Product2/2
  Compare To Constant/1 -> Product2/1
  Right/Left [1/0]/1 -> [RightLeft]
  [ExitingStance] -> Logical Operator/2
  [RightLeft] -> Logical Operator/1

== system vertical_smm_with_lqr_2d/Control/Behavior Control/Secondary Leg Behavior/Back//Front Motor PD ==
  Desired Position [rad] [back front] : Inport
  Desired Velocity [rad/s] [back front] : Inport  Port=2
  Desired Acceleration [rad/s^2] [back front] : Inport  Port=3
  Measured Position [rad] [back front] : Inport  Port=4
  Measured Velocity [rad/s] [back front] : Inport  Port=5
  Right/Left Leg [1/0] : Inport  Port=6
  Friction Compensation : Subsystem
  Product : Product
  Sum1 : Sum  Inputs=|++
  Sum2 : Sum  Inputs=|++
  Sum7 : Sum  Inputs=|+-
  Sum8 : Sum  Inputs=|+-
  Sum9 : Sum
  Switch : Switch  Criteria=u2 ~= 0
  kd : Gain  Gain=kd_motor
  kp : Gain  Gain=kp_motor
  left_inertias : Constant  Value=j_segments(3:4)
  reflected inertia : Constant  Value=j_motor
  right_inertias : Constant  Value=j_segments(1:2)
  Commanded Torque [Nm] [back front] : Outport
  wires:
  kp/1 -> Sum9/1
  Sum7/1 -> kp/1
  Measured Position [rad] [back front]/1 -> Sum7/2
  Sum9/1 -> Sum1/1
  Sum8/1 -> kd/1
  Desired Position [rad] [back front]/1 -> Sum7/1
  kd/1 -> Sum9/2
  Measured Velocity [rad/s] [back front]/1 -> Sum8/2
  Sum1/1 -> Sum2/1
  Desired Acceleration [rad/s^2] [back front]/1 -> Product/1
  Product/1 -> Sum1/2
  Right/Left Leg [1/0]/1 -> Friction Compensation/1(Right/Left [1/0]), Switch/2
  right_inertias/1 -> Switch/1
  left_inertias/1 -> Switch/3
  Sum2/1 -> Commanded Torque [Nm] [back front]/1
  Desired Velocity [rad/s] [back front]/1 -> Friction Compensation/2(Commanded Velocity [rad/s] [back front]), Sum8/1
  reflected inertia/1 -> Product/2

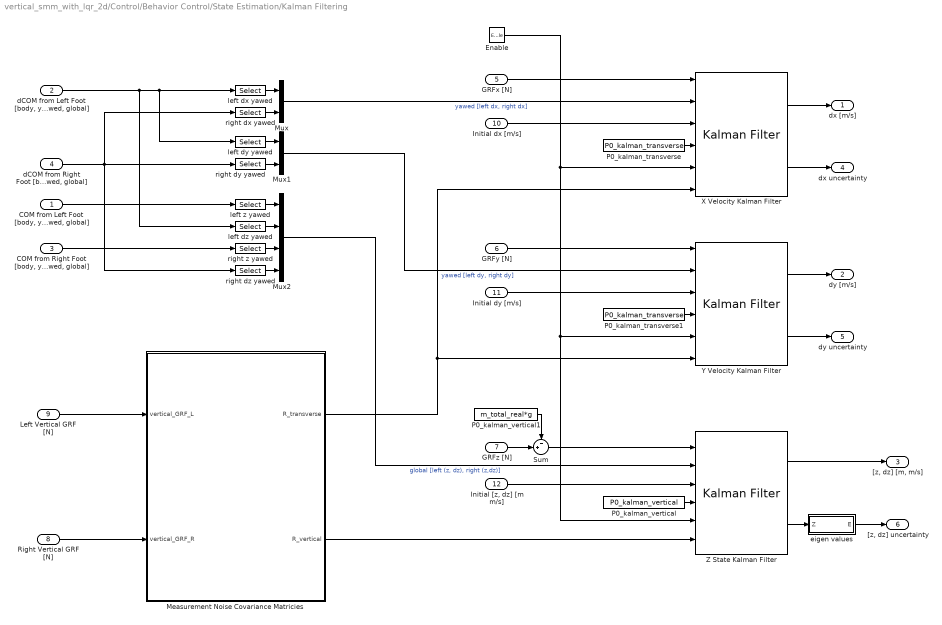
== system vertical_smm_with_lqr_2d/Control/Behavior Control/State Estimation/Kalman Filtering ==
  "COM from Left Foot [body, yawed, global]" : Inport  SampleTime=sample_time
  "dCOM from Left Foot [body, yawed, global]" : Inport  Port=2  SampleTime=sample_time
  "COM from Right Foot [body, yawed, global]" : Inport  Port=3  SampleTime=sample_time
  "dCOM from Right Foot [body, yawed, global]" : Inport  Port=4  SampleTime=sample_time
  GRFx [N] : Inport  Port=5  SampleTime=sample_time
  GRFy [N] : Inport  Port=6  SampleTime=sample_time
  GRFz [N] : Inport  Port=7  SampleTime=sample_time
  Right Vertical GRF [N] : Inport  Port=8  SampleTime=sample_time
  Left Vertical GRF [N] : Inport  Port=9  SampleTime=sample_time
  Initial dx [m/s] : Inport  Port=10  PortDimensions=1  SampleTime=sample_time
  Initial dy [m/s] : Inport  Port=11  PortDimensions=1  SampleTime=sample_time
  "Initial [z, dz] [m m/s]" : Inport  Port=12  PortDimensions=2  SampleTime=sample_time
  Enable : EnablePort  ShowOutputPort=on
  Measurement Noise Covariance Matricies : MATLAB Function  TreatAsAtomicUnit=on
  Mux : Mux  Inputs=2
  Mux1 : Mux  Inputs=2
  Mux2 : Mux
  P0_kalman_transverse : Constant  Value=P0_kalman_transverse
  P0_kalman_transverse1 : Constant  Value=P0_kalman_transverse
  P0_kalman_vertical : Constant  Value=P0_kalman_vertical
  P0_kalman_vertical1 : Constant  Value=m_total_real*g
  Sum : Sum  Inputs=-+|
  X Velocity Kalman Filter : ctrlSharedLib/Kalman Filter  TimeDomain=Discrete-Time  UseCurrentEstimator=on  ModelSource=Individual A, B, C, D matrices  ModelSourceVariable=A_kf  A=A_kalman_transverse  B=B_kalman_transverse  C=C_kalman_transverse  D=0  NumberOfStates=2  NumberOfInputs=1  NumberOfOutputs=2  InitialEstimateSource=Input port  X0=initial_dx_estimate  P0=P0_kalman_transverse  UseK=off  UseGH=on  NumberOfProcessNoiseInputs=1  G=G_kalman_transverse  TimeInvariantG=on  H=0  TimeInvariantH=on  Q=Q_kalman_GRF  TimeInvariantQ=on  R=1  TimeInvariantR=off  N=0  TimeInvariantN=on  AddInputPort=on  AddEnablePort=off  ExternalReset=Either  OutputEstimatedY=off  OutputP=on  Ts=sample_time
  Y Velocity Kalman Filter : ctrlSharedLib/Kalman Filter  TimeDomain=Discrete-Time  UseCurrentEstimator=on  ModelSource=Individual A, B, C, D matrices  ModelSourceVariable=A_kf  A=A_kalman_transverse  B=B_kalman_transverse  C=C_kalman_transverse  D=0  NumberOfStates=2  NumberOfInputs=1  NumberOfOutputs=2  InitialEstimateSource=Input port  X0=initial_dy_estimate  P0=P0_kalman_transverse  UseK=off  UseGH=on  NumberOfProcessNoiseInputs=1  G=G_kalman_transverse  TimeInvariantG=on  H=0  TimeInvariantH=on  Q=Q_kalman_GRF  TimeInvariantQ=on  R=1  TimeInvariantR=off  N=0  TimeInvariantN=on  AddInputPort=on  AddEnablePort=off  ExternalReset=Either  OutputEstimatedY=off  OutputP=on  Ts=sample_time
  Z State Kalman Filter : ctrlSharedLib/Kalman Filter  TimeDomain=Discrete-Time  UseCurrentEstimator=on  ModelSource=Individual A, B, C, D matrices  ModelSourceVariable=A_kf  A=A_kalman_vertical  B=B_kalman_vertical  C=C_kalman_vertical  D=0  NumberOfStates=2  NumberOfInputs=1  NumberOfOutputs=2  InitialEstimateSource=Input port  X0=[initial_z_estimate; initial_dz_estimate]  P0=P0_kalman_vertical  UseK=off  UseGH=on  NumberOfProcessNoiseInputs=1  G=G_kalman_vertical  TimeInvariantG=on  H=0  TimeInvariantH=on  Q=Q_kalman_GRF  TimeInvariantQ=on  R=1  TimeInvariantR=off  N=0  TimeInvariantN=on  AddInputPort=on  AddEnablePort=off  ExternalReset=Either  OutputEstimatedY=off  OutputP=on  Ts=sample_time
  eigen values : MATLAB Function  TreatAsAtomicUnit=on
  left dx yawed : Selector  InputPortWidth=9  Indices=[4]
  left dy yawed : Selector  InputPortWidth=9  Indices=[5]
  left dz yawed : Selector  InputPortWidth=9  Indices=[6]
  left z yawed : Selector  InputPortWidth=9  Indices=[6]
  right dx yawed : Selector  InputPortWidth=9  Indices=[4]
  right dy yawed : Selector  InputPortWidth=9  Indices=[5]
  right dz yawed : Selector  InputPortWidth=9  Indices=[6]
  right z yawed : Selector  InputPortWidth=9  Indices=[6]
  dx [m/s] : Outport
  dy [m/s] : Outport  Port=2
  "[z, dz] [m, m/s]" : Outport  Port=3
  dx uncertainty : Outport  Port=4
  dy uncertainty : Outport  Port=5
  "[z, dz] uncertainty" : Outport  Port=6
  wires:
  GRFy [N]/1 -> Y Velocity Kalman Filter/1
  Mux2/1 -> Z State Kalman Filter/2  "global [left (z, dz), right (z,dz)]"
  GRFx [N]/1 -> X Velocity Kalman Filter/1
  Measurement Noise Covariance Matricies/2(R_vertical) -> Z State Kalman Filter/6
  Measurement Noise Covariance Matricies/1(R_transverse) -> X Velocity Kalman Filter/6, Y Velocity Kalman Filter/6
  Mux1/1 -> Y Velocity Kalman Filter/2  "yawed [left dy, right dy]"
  Sum/1 -> Z State Kalman Filter/1
  Mux/1 -> X Velocity Kalman Filter/2  "yawed [left dx, right dx]"
  Right Vertical GRF [N]/1 -> Measurement Noise Covariance Matricies/2(vertical_GRF_R)
  Left Vertical GRF [N]/1 -> Measurement Noise Covariance Matricies/1(vertical_GRF_L)
  Z State Kalman Filter/1 -> "[z, dz] [m, m/s]"/1
  Y Velocity Kalman Filter/1 -> dy [m/s]/1
  X Velocity Kalman Filter/1 -> dx [m/s]/1
  "dCOM from Left Foot [body, yawed, global]"/1 -> left dy yawed/1, left dx yawed/1, left dz yawed/1
  left dx yawed/1 -> Mux/1
  "dCOM from Right Foot [body, yawed, global]"/1 -> right dx yawed/1, right dz yawed/1, right dy yawed/1
  right dx yawed/1 -> Mux/2
  left dy yawed/1 -> Mux1/1
  right dy yawed/1 -> Mux1/2
  left z yawed/1 -> Mux2/1
  right z yawed/1 -> Mux2/3
  left dz yawed/1 -> Mux2/2
  right dz yawed/1 -> Mux2/4
  "COM from Left Foot [body, yawed, global]"/1 -> left z yawed/1
  "COM from Right Foot [body, yawed, global]"/1 -> right z yawed/1
  P0_kalman_transverse/1 -> X Velocity Kalman Filter/4
  Initial dx [m/s]/1 -> X Velocity Kalman Filter/3
  P0_kalman_transverse1/1 -> Y Velocity Kalman Filter/4
  Initial dy [m/s]/1 -> Y Velocity Kalman Filter/3
  P0_kalman_vertical/1 -> Z State Kalman Filter/4
  "Initial [z, dz] [m m/s]"/1 -> Z State Kalman Filter/3
  GRFz [N]/1 -> Sum/2
  P0_kalman_vertical1/1 -> Sum/1
  Enable/1 -> Z State Kalman Filter/5, Y Velocity Kalman Filter/5, X Velocity Kalman Filter/5
  X Velocity Kalman Filter/2 -> dx uncertainty/1
  Y Velocity Kalman Filter/2 -> dy uncertainty/1
  Z State Kalman Filter/2 -> eigen values/1(Z)
  eigen values/1(E) -> "[z, dz] uncertainty"/1

== system vertical_smm_with_lqr_2d/Control/Behavior Control/State Estimation/Recursive Moving Average ==
  Velocity [m/s] : Inport
  Delay : Delay  DelayLength=velocity_avg_samples  InitialCondition=0  UseCircularBuffer=on  SampleTime=sample_time
  Gain : Gain  Gain=1/velocity_avg_samples
  Sum : Sum  Inputs=-++
  Unit Delay : UnitDelay  SampleTime=sample_time
  Average Velocity [m/s] : Outport
  wires:
  Unit Delay/1 -> Sum/3
  Gain/1 -> Average Velocity [m/s]/1
  Delay/1 -> Sum/1
  Sum/1 -> Gain/1, Unit Delay/1
  Velocity [m/s]/1 -> Sum/2, Delay/1

== system vertical_smm_with_lqr_2d/Control/Behavior Control/Primary Leg Behavior/Running/Circular Buffer ==
  Flight [1/0] : Inport
  Exiting Stance [1/0] : Inport  Port=2
  Hopping [1/0] : Inport  Port=3
  dX [m/s] : Inport  Port=4
  dY [m/s] : Inport  Port=5
  X Foot Correction [m] : Inport  Port=6
  Y Foot Correction [m] : Inport  Port=7
  target dX [m/s] : Inport  Port=8
  target dY [m/s] : Inport  Port=9
  Buffer : MATLAB Function  TreatAsAtomicUnit=on  SystemSampleTime=0.001
  Buffer1 : MATLAB Function  TreatAsAtomicUnit=on  SystemSampleTime=0.001
  Buffer2 : MATLAB Function  TreatAsAtomicUnit=on  SystemSampleTime=0.001
  Buffer3 : MATLAB Function  TreatAsAtomicUnit=on  SystemSampleTime=0.001
  Buffer4 : MATLAB Function  TreatAsAtomicUnit=on  SystemSampleTime=0.001
  Buffer5 : MATLAB Function  TreatAsAtomicUnit=on  SystemSampleTime=0.001
  Buffer6 : MATLAB Function  TreatAsAtomicUnit=on  SystemSampleTime=0.001
  Buffer7 : MATLAB Function  TreatAsAtomicUnit=on  SystemSampleTime=0.001
  Demux : Demux  Outputs=6
  Detect Decrease : simulink/Logic and Bit Operations/Detect Decrease  vinit=0.0  InputProcessing=Inherited  OutDataTypeStr=boolean
  Enabled on Touchdown : Subsystem  TreatAsAtomicUnit=on
  Logical Operator : Logic  AllPortsSameDT=off  OutDataTypeStr=boolean
  Mux : Mux  Inputs=6
  buffer size5 : Constant  Value=recorded_steps
  "dX Touchdown History " : Outport
  X Foot Correction History : Outport  Port=2
  dX Takeoff History : Outport  Port=3
  "dY Touchdown History " : Outport  Port=4
  Y Foot Correction History : Outport  Port=5
  dY Takeoff History : Outport  Port=6
  target dX History : Outport  Port=7
  target dY History : Outport  Port=8
  wires:
  Buffer/1(buffer) -> "dX Touchdown History "/1
  Detect Decrease/1 -> Enabled on Touchdown/Enable
  Buffer1/1(buffer) -> X Foot Correction History/1
  Buffer2/1(buffer) -> dX Takeoff History/1
  Demux/1 -> Buffer/1(data)
  Demux/3 -> Buffer1/1(data)
  X Foot Correction [m]/1 -> Mux/3
  Buffer3/1(buffer) -> "dY Touchdown History "/1
  Buffer4/1(buffer) -> Y Foot Correction History/1
  Demux/2 -> Buffer3/1(data)
  Buffer5/1(buffer) -> dY Takeoff History/1
  Y Foot Correction [m]/1 -> Mux/4
  Demux/4 -> Buffer4/1(data)
  target dX [m/s]/1 -> Mux/5
  Buffer6/1(buffer) -> target dX History/1
  Buffer7/1(buffer) -> target dY History/1
  buffer size5/1 -> Buffer2/3(buffer_size), Buffer/3(buffer_size), Buffer7/3(buffer_size), Buffer6/3(buffer_size), Buffer4/3(buffer_size), Buffer1/3(buffer_size), Buffer3/3(buffer_size), Buffer5/3(buffer_size)
  Demux/6 -> Buffer7/1(data)
  Demux/5 -> Buffer6/1(data)
  target dY [m/s]/1 -> Mux/6
  Exiting Stance [1/0]/1 -> Buffer/2(trigger), Buffer7/2(trigger), Buffer6/2(trigger), Buffer4/2(trigger), Buffer1/2(trigger), Buffer3/2(trigger), Buffer2/2(trigger), Buffer5/2(trigger)
  Hopping [1/0]/1 -> Logical Operator/1
  dY [m/s]/1 -> Buffer5/1(data), Mux/2
  dX [m/s]/1 -> Buffer2/1(data), Mux/1
  Flight [1/0]/1 -> Logical Operator/2
  Logical Operator/1 -> Detect Decrease/1
  Mux/1 -> Enabled on Touchdown/1(In)
  Enabled on Touchdown/1(Out) -> Demux/1

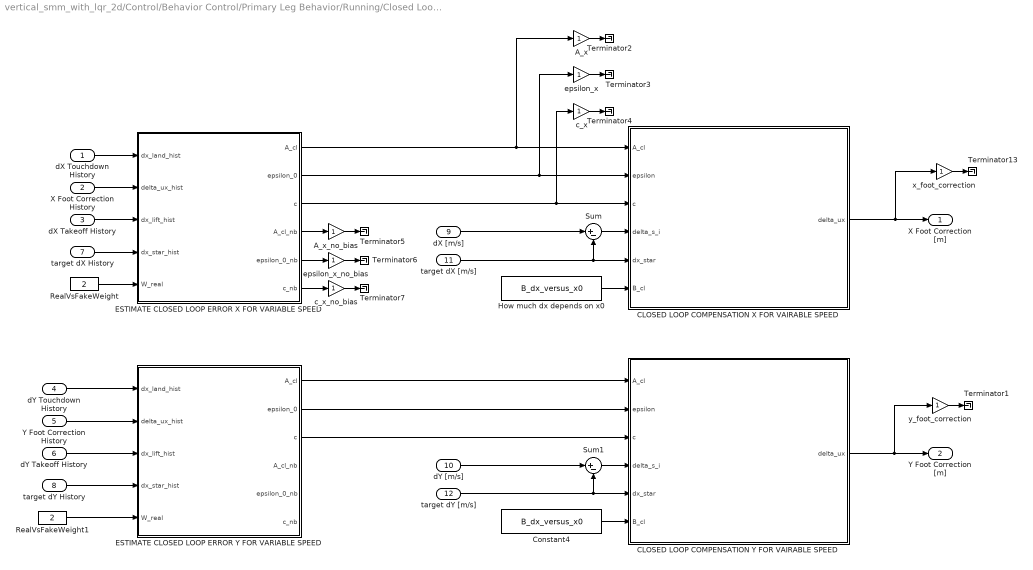
== system vertical_smm_with_lqr_2d/Control/Behavior Control/Primary Leg Behavior/Running/Closed Loop Compensation ==
  dX Touchdown History : Inport
  X Foot Correction History : Inport  Port=2
  dX Takeoff History : Inport  Port=3
  dY Touchdown History : Inport  Port=4
  Y Foot Correction History : Inport  Port=5
  dY Takeoff History : Inport  Port=6
  target dX History : Inport  Port=7
  target dY History : Inport  Port=8
  dX [m/s] : Inport  Port=9
  dY [m/s] : Inport  Port=10
  target dX [m/s] : Inport  Port=11
  "target dY [m/s] " : Inport  Port=12
  A_x : Gain
  A_x_no_bias : Gain
  CLOSED LOOP COMPENSATION X FOR VAIRABLE SPEED : MATLAB Function  TreatAsAtomicUnit=on
  CLOSED LOOP COMPENSATION Y FOR VAIRABLE SPEED : MATLAB Function  TreatAsAtomicUnit=on
  Constant4 : Constant  Value=B_dx_versus_x0
  ESTIMATE CLOSED LOOP ERROR X FOR VARIABLE SPEED : MATLAB Function  TreatAsAtomicUnit=on
  ESTIMATE CLOSED LOOP ERROR Y FOR VARIABLE SPEED : MATLAB Function  TreatAsAtomicUnit=on
  How much dx depends on x0 : Constant  Value=B_dx_versus_x0
  RealVsFakeWeight : Constant  Value=2
  RealVsFakeWeight1 : Constant  Value=2
  Sum : Sum  Inputs=|+-
  Sum1 : Sum  Inputs=|+-
  Terminator{1..7,13} (8 alike) : Terminator
  c_x : Gain
  c_x_no_bias : Gain
  epsilon_x : Gain
  epsilon_x_no_bias : Gain
  x_foot_correction : Gain
  y_foot_correction : Gain
  X Foot Correction [m] : Outport
  Y Foot Correction [m] : Outport  Port=2
  wires:
  RealVsFakeWeight1/1 -> ESTIMATE CLOSED LOOP ERROR Y FOR VARIABLE SPEED/5(W_real)
  Constant4/1 -> CLOSED LOOP COMPENSATION Y FOR VAIRABLE SPEED/6(B_cl)
  "target dY [m/s] "/1 -> Sum1/2, CLOSED LOOP COMPENSATION Y FOR VAIRABLE SPEED/5(dx_star)
  ESTIMATE CLOSED LOOP ERROR Y FOR VARIABLE SPEED/3(c) -> CLOSED LOOP COMPENSATION Y FOR VAIRABLE SPEED/3(c)
  ESTIMATE CLOSED LOOP ERROR Y FOR VARIABLE SPEED/2(epsilon_0) -> CLOSED LOOP COMPENSATION Y FOR VAIRABLE SPEED/2(epsilon)
  ESTIMATE CLOSED LOOP ERROR Y FOR VARIABLE SPEED/1(A_cl) -> CLOSED LOOP COMPENSATION Y FOR VAIRABLE SPEED/1(A_cl)
  target dY History/1 -> ESTIMATE CLOSED LOOP ERROR Y FOR VARIABLE SPEED/4(dx_star_hist)
  Y Foot Correction History/1 -> ESTIMATE CLOSED LOOP ERROR Y FOR VARIABLE SPEED/2(delta_ux_hist)
  dY Takeoff History/1 -> ESTIMATE CLOSED LOOP ERROR Y FOR VARIABLE SPEED/3(dx_lift_hist)
  dY [m/s]/1 -> Sum1/1
  RealVsFakeWeight/1 -> ESTIMATE CLOSED LOOP ERROR X FOR VARIABLE SPEED/5(W_real)
  How much dx depends on x0/1 -> CLOSED LOOP COMPENSATION X FOR VAIRABLE SPEED/6(B_cl)
  Sum/1 -> CLOSED LOOP COMPENSATION X FOR VAIRABLE SPEED/4(delta_s_i)
  target dX [m/s]/1 -> Sum/2, CLOSED LOOP COMPENSATION X FOR VAIRABLE SPEED/5(dx_star)
  ESTIMATE CLOSED LOOP ERROR X FOR VARIABLE SPEED/3(c) -> CLOSED LOOP COMPENSATION X FOR VAIRABLE SPEED/3(c), c_x/1
  ESTIMATE CLOSED LOOP ERROR X FOR VARIABLE SPEED/2(epsilon_0) -> CLOSED LOOP COMPENSATION X FOR VAIRABLE SPEED/2(epsilon), epsilon_x/1
  ESTIMATE CLOSED LOOP ERROR X FOR VARIABLE SPEED/1(A_cl) -> CLOSED LOOP COMPENSATION X FOR VAIRABLE SPEED/1(A_cl), A_x/1
  target dX History/1 -> ESTIMATE CLOSED LOOP ERROR X FOR VARIABLE SPEED/4(dx_star_hist)
  X Foot Correction History/1 -> ESTIMATE CLOSED LOOP ERROR X FOR VARIABLE SPEED/2(delta_ux_hist)
  dX Takeoff History/1 -> ESTIMATE CLOSED LOOP ERROR X FOR VARIABLE SPEED/3(dx_lift_hist)
  dX Touchdown History/1 -> ESTIMATE CLOSED LOOP ERROR X FOR VARIABLE SPEED/1(dx_land_hist)
  dX [m/s]/1 -> Sum/1
  dY Touchdown History/1 -> ESTIMATE CLOSED LOOP ERROR Y FOR VARIABLE SPEED/1(dx_land_hist)
  Sum1/1 -> CLOSED LOOP COMPENSATION Y FOR VAIRABLE SPEED/4(delta_s_i)
  CLOSED LOOP COMPENSATION X FOR VAIRABLE SPEED/1(delta_ux) -> x_foot_correction/1, X Foot Correction [m]/1
  x_foot_correction/1 -> Terminator13/1
  CLOSED LOOP COMPENSATION Y FOR VAIRABLE SPEED/1(delta_ux) -> y_foot_correction/1, Y Foot Correction [m]/1
  y_foot_correction/1 -> Terminator1/1
  A_x/1 -> Terminator2/1
  epsilon_x/1 -> Terminator3/1
  c_x/1 -> Terminator4/1
  ESTIMATE CLOSED LOOP ERROR X FOR VARIABLE SPEED/6(c_nb) -> c_x_no_bias/1
  ESTIMATE CLOSED LOOP ERROR X FOR VARIABLE SPEED/5(epsilon_0_nb) -> epsilon_x_no_bias/1
  ESTIMATE CLOSED LOOP ERROR X FOR VARIABLE SPEED/4(A_cl_nb) -> A_x_no_bias/1
  A_x_no_bias/1 -> Terminator5/1
  epsilon_x_no_bias/1 -> Terminator6/1
  c_x_no_bias/1 -> Terminator7/1
